simulink library "mach_lib"  (Simulink 6.3)
undefined symbols (not defined in the file): accel_cmd, aero_surf_qbar_off, aero_surf_qbar_on, altitude_stop, angular_rate_stop, att_cmd_select, att_trim_IC, att_type, att_type_numbers, bb_ellipsoid, bb_params, chi_trim_IC, command_time, compute_all_rate_cols, compute_all_vel_cols, constants, cosA, da_trim_IC, de_trim_IC, DiscIntNeverNeededParam, dr_trim_IC, dtsim, E_rwy, E_trim_IC, Ed_cmd, Ed_trim_IC, energy_stop, eow_boundary, full_surf_llim, full_surf_ulim, gain_var_struct, gam_cmd_descent, gam_cmd_preflare, gamdot_cmd_descent, gamdot_cmd_flare, gamdot_cmd_preflare, gamma_trim_IC, h_trim_IC, hd_cmd, hd_trim_IC, ideal_vel_Kb, integrate_start_time_sim, integrate_state_sim, llim, MACH, MACH_att_fb, MACH_gain_mat, MACH_mass_IC, MACH_pos_IC, MACH_pqr_Bmat_IC, MACH_pqr_IC, MACH_pqr_u_IC, MACH_quat_IC, MACH_throttle_IC, MACH_U_nom_IC, MACH_vel_Bmat_IC, MACH_vel_cvdnom_IC, MACH_vel_IC, MACH_vel_uold_IC, max_chi_cmd ... (+67)
libraries: simulink x75, mach_lib x27, utility_lib x25, model_lib x7, models x6
(part 5 of 6)

== system mach_lib/claw_main/state est/wind estimator/wind estimate ==
  note: Note: wind estimator used to assume sensed accel
      | at some (modeled) sensor location offset.
      |  Current code assumes sensed accel at CG.
  dircos : Inport
  x : Inport  Port=2
  xdot : Inport  Port=3
  model_accels_cg : Inport  Port=4
  sensed_accels_cg : Inport  Port=5
  wind_est_sw : Inport  Port=6
  Bus Creator : BusCreator  Inputs=5
  Bus Selector : BusSelector  OutputSignals=uvw
  Data Type Conversion : DataTypeConversion  OutDataTypeMode=double  SaturateOnIntegerOverflow=on  RndMeth=Zero
  Discrete-Time Integrator : DiscreteIntegrator  SampleTime=-1  ICPrevOutput=DiscIntNeverNeededParam  ICPrevScaledInput=DiscIntNeverNeededParam
  Gain : Gain  Gain=MACH.est_w_Kuvw  SaturateOnIntegerOverflow=on
  Gain1 : Gain  Orientation=left  Gain=MACH.est_w_Kaw  SaturateOnIntegerOverflow=on
  Math Function : Math  Operator=transpose  SaturateOnIntegerOverflow=on
  Product : Product  Multiplication=Matrix(*)  SaturateOnIntegerOverflow=on
  Product1 : Product  Orientation=left  Multiplication=Matrix(*)  SaturateOnIntegerOverflow=on
  Product2 : Product  SaturateOnIntegerOverflow=on
  Product3 : Product  SaturateOnIntegerOverflow=on
  Reshape : simulink/Math Operations/Reshape  OutputDimensionality=Customize  OutputDimensions=[3,3]
  Sum : Sum  Inputs=++|  SaturateOnIntegerOverflow=on  InputSameDT=on
  Sum1 : Sum  Inputs=|+-  SaturateOnIntegerOverflow=on  InputSameDT=on
  Sum2 : Sum  Inputs=-+|  SaturateOnIntegerOverflow=on
  Sum3 : Sum  Orientation=left  Inputs=-+|  SaturateOnIntegerOverflow=on
  Sum4 : Sum  Inputs=|++  SaturateOnIntegerOverflow=on  InputSameDT=on
  Unit Delay1 : UnitDelay  Orientation=left  X0=zeros(3,1)  SampleTime=-1
  rate and  position limits : Subsystem
  uvw : Selector  Elements=MACH.uvw_idx  InputPortWidth=MACH.num_x
  w_est : Outport
  w_est_debug : Outport  Port=2
  wires:
  model_accels_cg/1 -> [accels], Sum1/2
  Bus Creator/1 -> w_est_debug/1
  [accels] -> Bus Creator/5  "accels"
  [uvw_rw_est] -> Bus Creator/4  "uvw_rw_est"
  [uvw_wind] -> Bus Creator/3  "uvw_wind"
  Data Type Conversion/1 -> Product3/1, Product2/1
  Unit Delay1/1 -> Sum4/2
  Product3/1 -> Sum4/1
  Sum4/1 -> Discrete-Time Integrator/1
  wind_est_sw/1 -> Data Type Conversion/1
  Product2/1 -> Bus Creator/1, Sum3/2, w_est/1  "w_est"
  Sum3/1 -> Bus Creator/2, Product1/2  "NED_wind_ex"
  Product1/1 -> Gain1/1
  rate and  position limits/1(w_est_lim) -> Product2/2
  x/1 -> Bus Selector/1
  uvw/1 -> Sum/1
  xdot/1 -> uvw/1
  Gain1/1 -> Unit Delay1/1
  Sum2/1 -> [uvw_wind], Product/2
  Math Function/1 -> Product/1
  Product/1 -> rate and  position limits/1(w_est), Sum3/1
  Reshape/1 -> Product1/1, Math Function/1
  dircos/1 -> Reshape/1
  Bus Selector/1 -> Sum2/1  "<uvw>"
  Gain/1 -> Sum/2
  Sum/1 -> Product3/2
  Sum1/1 -> Gain/1
  sensed_accels_cg/1 -> Sum1/1
  Discrete-Time Integrator/1 -> [uvw_rw_est], Sum2/2

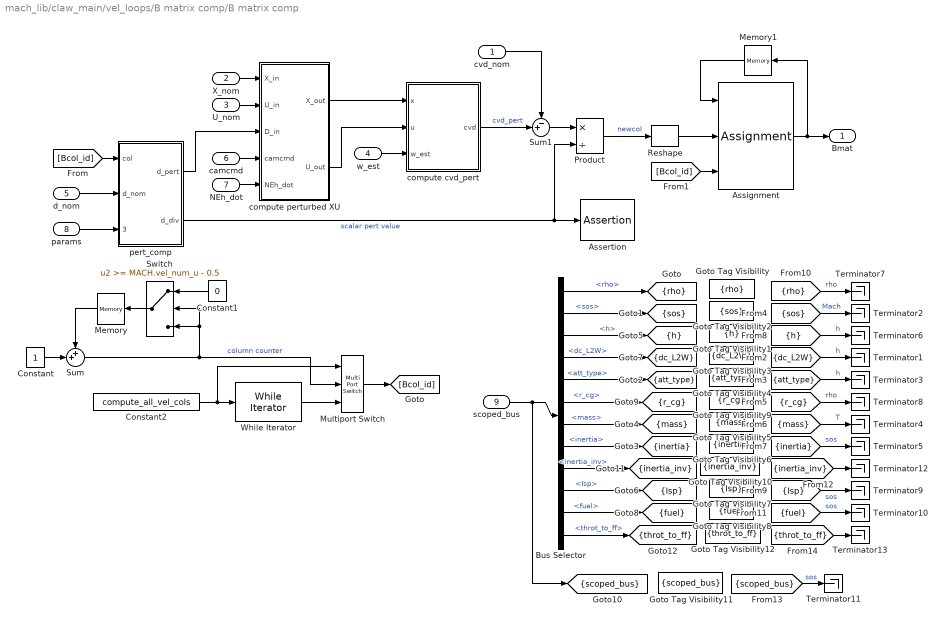
== system mach_lib/claw_main/vel_loops/B matrix comp/B matrix comp ==
  cvd_nom : Inport
  X_nom : Inport  Port=2
  U_nom : Inport  Port=3
  w_est : Inport  Port=4
  d_nom : Inport  Port=5
  camcmd : Inport  Port=6
  NEh_dot : Inport  Port=7
  params : Inport  Port=8
  scoped_bus : Inport  Port=9
  Assertion : Assertion
  Assignment : Assignment  InputType=Matrix  Rows=-1  ColumnSrc=External
  Bus Selector : BusSelector  OutputSignals=atmos_env.rho,atmos_env.sos,atmos_env.h,dc_L2W,att_type,mass_props.r_cg,mass_props.mass,mass_props.inertia,mass_props.inertia_inv,mass_props.Isp,mass_props.fuel,mass_props.throt_to_ff
  Constant : Constant
  Constant1 : Constant  Orientation=left  Value=0
  Constant2 : Constant  Value=compute_all_vel_cols
  Goto Tag Visibility : GotoTagVisibility  GotoTag=rho
  Goto Tag Visibility1 : GotoTagVisibility  GotoTag=h
  Goto Tag Visibility10 : GotoTagVisibility  GotoTag=inertia_inv
  Goto Tag Visibility11 : GotoTagVisibility  GotoTag=scoped_bus
  Goto Tag Visibility12 : GotoTagVisibility  GotoTag=throt_to_ff
  Goto Tag Visibility2 : GotoTagVisibility  GotoTag=sos
  Goto Tag Visibility3 : GotoTagVisibility  GotoTag=dc_L2W
  Goto Tag Visibility4 : GotoTagVisibility  GotoTag=att_type
  Goto Tag Visibility5 : GotoTagVisibility  GotoTag=mass
  Goto Tag Visibility6 : GotoTagVisibility  GotoTag=inertia
  Goto Tag Visibility7 : GotoTagVisibility  GotoTag=Isp
  Goto Tag Visibility8 : GotoTagVisibility  GotoTag=fuel
  Goto Tag Visibility9 : GotoTagVisibility  GotoTag=r_cg
  Memory : Memory  Orientation=left  InheritSampleTime=on
  Memory1 : Memory  Orientation=left  X0=MACH_vel_Bmat_IC  InheritSampleTime=on
  Multiport Switch : MultiPortSwitch  Inputs=2  zeroidx=on
  Product : Product  Inputs=*/  SaturateOnIntegerOverflow=on  InputSameDT=on
  Reshape : simulink/Math Operations/Reshape  OutputDimensionality=Column vector  OutputDimensions=[1,1]
  Sum : Sum  Inputs=++|  SaturateOnIntegerOverflow=on  InputSameDT=on
  Sum1 : Sum  Inputs=-+|  SaturateOnIntegerOverflow=on  InputSameDT=on
  Switch : Switch  Orientation=left  Threshold=MACH.vel_num_u - 0.5  SaturateOnIntegerOverflow=on  InputSameDT=on
  Terminator{1..13} (13 alike) : Terminator
  While Iterator : WhileIterator  MaxIters=MACH.vel_num_u  WhileBlockType=do-while  ShowIterationPort=on
  compute cvd_pert : Subsystem
  compute perturbed XU : Subsystem
  pert_comp : Subsystem
  Bmat : Outport
  tag scope: Isp=scoped, att_type=scoped, dc_L2W=scoped, fuel=scoped, h=scoped, inertia=scoped, inertia_inv=scoped, mass=scoped, r_cg=scoped, rho=scoped, scoped_bus=scoped, sos=scoped, throt_to_ff=scoped
  wires:
  [throt_to_ff] -> Terminator13/1
  Bus Selector/12 -> [throt_to_ff]  "<throt_to_ff>"
  [scoped_bus] -> Terminator11/1  "sos"
  Bus Selector/9 -> [inertia_inv]  "<inertia_inv>"
  [inertia_inv] -> Terminator12/1
  cvd_nom/1 -> Sum1/1
  compute cvd_pert/1(cvd) -> Sum1/2  "cvd_pert"
  Bus Selector/11 -> [fuel]  "<fuel>"
  [fuel] -> Terminator10/1  "sos"
  Bus Selector/10 -> [Isp]  "<Isp>"
  [Isp] -> Terminator9/1  "sos"
  Bus Selector/8 -> [inertia]  "<inertia>"
  Bus Selector/7 -> [mass]  "<mass>"
  Bus Selector/6 -> [r_cg]  "<r_cg>"
  [inertia] -> Terminator5/1  "sos"
  [mass] -> Terminator4/1  "T"
  [r_cg] -> Terminator8/1  "rho"
  Bus Selector/5 -> [att_type]  "<att_type>"
  [att_type] -> Terminator3/1  "h"
  Multiport Switch/1 -> [Bcol_id]
  Constant/1 -> Sum/2
  Memory/1 -> Sum/1
  Switch/1 -> Memory/1
  Sum/1 -> Multiport Switch/2, Switch/2, Switch/3  "column counter"
  Constant1/1 -> Switch/1
  While Iterator/1 -> Multiport Switch/3
  Constant2/1 -> While Iterator/1, Multiport Switch/1
  Bus Selector/4 -> [dc_L2W]  "<dc_L2W>"
  [dc_L2W] -> Terminator1/1  "h"
  Bus Selector/3 -> [h]  "<h>"
  Bus Selector/2 -> [sos]  "<sos>"
  Bus Selector/1 -> [rho]  "<rho>"
  [h] -> Terminator6/1  "h"
  [sos] -> Terminator2/1  "Mach"
  [rho] -> Terminator7/1  "rho"
  scoped_bus/1 -> [scoped_bus], Bus Selector/1
  Memory1/1 -> Assignment/1
  compute perturbed XU/2(U_out) -> compute cvd_pert/2(u)
  params/1 -> pert_comp/3(params)
  compute perturbed XU/1(X_out) -> compute cvd_pert/1(x)
  NEh_dot/1 -> compute perturbed XU/5(NEh_dot)
  camcmd/1 -> compute perturbed XU/4(camcmd)
  w_est/1 -> compute cvd_pert/3(w_est)
  pert_comp/1(d_pert) -> compute perturbed XU/3(D_in)
  pert_comp/2(d_div) -> Assertion/1, Product/2  "scalar pert value"
  d_nom/1 -> pert_comp/2(d_nom)
  [Bcol_id] -> pert_comp/1(col)
  Assignment/1 -> Memory1/1, Bmat/1
  Reshape/1 -> Assignment/2
  [Bcol_id] -> Assignment/3
  Sum1/1 -> Product/1
  Product/1 -> Reshape/1  "newcol"
  X_nom/1 -> compute perturbed XU/1(X_in)
  U_nom/1 -> compute perturbed XU/2(U_in)

== system mach_lib/claw_main/vel_loops/B matrix comp/compute cvd_nom ==
  note: Note: this computation of NEh accelerations
      | assumes that pqr = 0
  x : Inport
  u : Inport  Port=2
  w_est : Inport  Port=3
  Bus Selector : BusSelector  OutputSignals=dircos
  Gain : Gain  Gain=[1 1 -1]  SaturateOnIntegerOverflow=on
  Math Function : Math  Operator=transpose  SaturateOnIntegerOverflow=on
  Product : Product  Multiplication=Matrix(*)  SaturateOnIntegerOverflow=on  InputSameDT=on
  Reshape : simulink/Math Operations/Reshape  OutputDimensionality=Customize  OutputDimensions=[3,3]
  cl model : models/datcom-obac
  uvw_dot : Selector  Elements=MACH.uvw_idx  InputPortWidth=MACH.num_x
  cvd : Outport
  wires:
  cl model/2 -> Bus Selector/1
  cl model/1 -> uvw_dot/1
  w_est/1 -> cl model/3
  u/1 -> cl model/2
  Bus Selector/1 -> Reshape/1  "<dircos>"
  Gain/1 -> cvd/1
  Product/1 -> Gain/1
  Math Function/1 -> Product/1
  Reshape/1 -> Math Function/1
  x/1 -> cl model/1
  uvw_dot/1 -> Product/2

== system mach_lib/claw_main/vel_loops/B matrix comp/compute nominal XU ==
  X_in : Inport
  U_in : Inport  Port=2
  D_in : Inport  Port=3
  camcmd : Inport  Port=4
  NEh_dot : Inport  Port=5
  Assignment1 : Assignment  Elements=MACH.throttle_idx  OutputInitialize=Initialize using input (U1)
  Assignment2 : Assignment  Elements=[ MACH.quat_idx MACH.uvw_idx]  OutputInitialize=Initialize using input (U1)
  Demux1 : Demux  Outputs=[ 2 MACH.num_u_throt ]
  Gain : Gain  Gain=[1 1 -1]  SaturateOnIntegerOverflow=on
  Mux : Mux  Inputs=[ 2 1 ]
  Mux1 : Mux  Inputs=2
  Product1 : Product  Multiplication=Matrix(*)  SaturateOnIntegerOverflow=on
  Reshape1 : simulink/Math Operations/Reshape  OutputDimensionality=Customize  OutputDimensions=[3,3]
  Selector1 : Selector  Elements=MACH.quat_idx  InputPortWidth=MACH.num_x
  att2dc : utility_lib/att2dc
  dc2e_ref : utility_lib/dc2e_ref
  X_out : Outport
  U_out : Outport  Port=2
  wires:
  Mux1/1 -> Assignment2/2
  Product1/1 -> Mux1/2  "uvw"
  Selector1/1 -> dc2e_ref/2
  Gain/1 -> Product1/2  "NED_dot"
  dc2e_ref/1 -> Mux1/1  "e"
  att2dc/1 -> dc2e_ref/1, Reshape1/1
  Assignment2/1 -> X_out/1
  Reshape1/1 -> Product1/1
  NEh_dot/1 -> Gain/1
  Demux1/1 -> Mux/1
  camcmd/1 -> Mux/2
  Assignment1/1 -> U_out/1
  X_in/1 -> Selector1/1, Assignment2/1
  U_in/1 -> Assignment1/1
  D_in/1 -> Demux1/1
  Demux1/2 -> Assignment1/2  "throttle"
  Mux/1 -> att2dc/1

== system mach_lib/claw_main/vel_loops/convert accel_cmd to NED_dd_cmd/NED_dd cmd ==
  NEH_dd_cmd_in : Inport
  Action Port : ActionPort
  NEh_dd_cmd : Outport  InitialOutput=zeros(3,1)
  wires:
  NEH_dd_cmd_in/1 -> NEh_dd_cmd/1

== system mach_lib/claw_main/vel_loops/convert accel_cmd to NED_dd_cmd/vchigam_dot cmd ==
  vchigam_dot_cmd : Inport
  NEh_d : Inport  Port=2
  Action Port : ActionPort
  Math Function : Math  Operator=transpose  SaturateOnIntegerOverflow=on
  Product2 : Product  Multiplication=Matrix(*)  RndMeth=Zero
  Reshape1 : simulink/Math Operations/Reshape  OutputDimensionality=Customize  OutputDimensions=[3 3]
  convert to NED_d : Gain  Gain=[1 1 -1]
  convert to NEh_dd : Gain  Gain=[1 1 -1]
  polar to cart : Subsystem
  vec2dc : utility_lib/vec2dc
  NEh_dd_cmd : Outport  InitialOutput=zeros(3,1)
  wires:
  vec2dc/2 -> polar to cart/1(scaling_info)
  vchigam_dot_cmd/1 -> polar to cart/2(vchigam_dot_cmd)
  Math Function/1 -> Product2/1
  convert to NEh_dd/1 -> NEh_dd_cmd/1
  Product2/1 -> convert to NEh_dd/1
  NEh_d/1 -> convert to NED_d/1
  polar to cart/1(along_dd;cross_dd;vert_dd) -> Product2/2
  convert to NED_d/1 -> vec2dc/1
  Reshape1/1 -> Math Function/1
  vec2dc/1 -> Reshape1/1

== system mach_lib/claw_main/vel_loops/set di params/att limits ==
  uvw : Inport
  Bus Creator : BusCreator
  Constant : Constant  Value=MACH.vel_att_ulim  VectorParams1D=off
  Constant1 : Constant  Value=MACH.vel_att_lrlim
  Constant2 : Constant  Value=MACH.vel_att_urlim
  Constant3 : Constant  Value=MACH.az_ulim
  Constant7 : Constant  Value=MACH.vel_att_llim  VectorParams1D=off
  Constant8 : Constant  Value=MACH.az_llim
  Reshape1 : simulink/Math Operations/Reshape  OutputDimensionality=1-D array  OutputDimensions=[1,1]
  Reshape3 : simulink/Math Operations/Reshape  OutputDimensionality=1-D array  OutputDimensions=[1,1]
  Selector1 : Selector  InputType=Matrix  Elements=[1 3]  RowSrc=External  Columns=-1  InputPortWidth=3
  Selector2 : Selector  InputType=Matrix  Elements=[1 3]  RowSrc=External  Columns=-1  InputPortWidth=3
  velocity based angular rate llim : mach_lib/velocity based angular rate limit  q_idx=2
  velocity based angular rate ulim : mach_lib/velocity based angular rate limit  q_idx=2
  att_limits : Outport
  wires:
  Bus Creator/1 -> att_limits/1
  velocity based angular rate llim/1 -> Bus Creator/4  "att_lrlim"
  velocity based angular rate ulim/1 -> Bus Creator/3  "att_urlim"
  uvw/1 -> velocity based angular rate llim/3, velocity based angular rate ulim/3
  Constant3/1 -> velocity based angular rate llim/2
  Constant1/1 -> velocity based angular rate llim/1
  Constant8/1 -> velocity based angular rate ulim/2
  Constant2/1 -> velocity based angular rate ulim/1
  Reshape3/1 -> Bus Creator/2  "att_llim"
  Reshape1/1 -> Bus Creator/1  "att_ulim"
  Selector2/1 -> Reshape3/1
  Selector1/1 -> Reshape1/1
  Constant7/1 -> Selector2/1
  Constant/1 -> Selector1/1
  [att_type] -> Selector2/2, Selector1/2

== system mach_lib/claw_main/vel_loops/set di params/combine limits ==
  att_limits : Inport
  throt_limits : Inport  Port=2
  Bus Creator : BusCreator
  Bus Selector : BusSelector  OutputSignals=att_ulim,att_llim,att_urlim,att_lrlim
  Bus Selector1 : BusSelector  OutputSignals=throt_ulim,throt_llim,throt_urlim,throt_lrlim
  Mux{,1..3} (4 alike) : Mux  Inputs=2
  vel_u_limits : Outport
  wires:
  Bus Creator/1 -> vel_u_limits/1
  Mux3/1 -> Bus Creator/4  "u_lrlim"
  Mux2/1 -> Bus Creator/3  "u_urlim"
  Mux1/1 -> Bus Creator/2  "u_llim"
  Mux/1 -> Bus Creator/1  "u_ulim"
  Bus Selector1/4 -> Mux3/2  "<throt_lrlim>"
  Bus Selector1/3 -> Mux2/2  "<throt_urlim>"
  Bus Selector1/2 -> Mux1/2  "<throt_llim>"
  Bus Selector1/1 -> Mux/2  "<throt_ulim>"
  Bus Selector/4 -> Mux3/1  "<att_lrlim>"
  Bus Selector/3 -> Mux2/1  "<att_urlim>"
  Bus Selector/2 -> Mux1/1  "<att_llim>"
  Bus Selector/1 -> Mux/1  "<att_ulim>"
  throt_limits/1 -> Bus Selector1/1
  att_limits/1 -> Bus Selector/1

== system mach_lib/claw_main/vel_loops/set di params/compute dc_fltpath ==
  NEh_dot_fltpath : Inport
  Gain : Gain  Gain=repmat([1 1 -1],3,1)
  Gain1 : Gain  Gain=[1 1 -1]
  Reshape : simulink/Math Operations/Reshape  OutputDimensionality=Customize  OutputDimensions=[3 3]
  Terminator : Terminator
  vec2dc : utility_lib/vec2dc
  dc_fltpath : Outport
  wires:
  NEh_dot_fltpath/1 -> Gain1/1
  Gain/1 -> dc_fltpath/1
  vec2dc/2 -> Terminator/1
  Gain1/1 -> vec2dc/1
  Reshape/1 -> Gain/1
  vec2dc/1 -> Reshape/1

== system mach_lib/claw_main/vel_loops/set di params/throttle limits ==
  full_surf : Inport
  throt_old : Inport  Port=2
  Bus Creator : BusCreator
  Bus Selector1 : BusSelector  OutputSignals=full_surf_ulim,full_surf_llim,full_surf_urlim,full_surf_lrlim
  Selector{1..2,5..6} (4 alike) : Selector  Elements=MACH.throttle_idx  InputPortWidth=MACH.num_u
  rate limit limits : mach_lib/rate limit limits  ulim=MACH.vel_throt_ulim  llim=MACH.vel_throt_llim
  throt_limits : Outport
  wires:
  Selector2/1 -> Bus Creator/4, rate limit limits/5  "throt_lrlim"
  Selector1/1 -> Bus Creator/3, rate limit limits/4  "throt_urlim"
  Bus Selector1/4 -> Selector2/1  "<full_surf_lrlim>"
  Bus Selector1/3 -> Selector1/1  "<full_surf_urlim>"
  rate limit limits/2 -> Bus Creator/2  "throt_llim"
  rate limit limits/1 -> Bus Creator/1  "throt_ulim"
  Bus Creator/1 -> throt_limits/1
  Selector6/1 -> rate limit limits/3
  Selector5/1 -> rate limit limits/2
  throt_old/1 -> rate limit limits/1
  full_surf/1 -> Bus Selector1/1
  Bus Selector1/2 -> Selector6/1  "<full_surf_llim>"
  Bus Selector1/1 -> Selector5/1  "<full_surf_ulim>"

== system mach_lib/control input/form control input/select command/att cmd select ==
  cmd_bus : Inport
  Bus Selector1 : BusSelector  OutputSignals=att1_cmd,att2_cmd,att3_cmd,throttle_cmd  OutputAsBus=on
  Bus Selector2 : BusSelector  OutputSignals=att_cmd
  Switch : Switch  Threshold=0.5
  use_cam_rate_cmd1 : Constant  Value=att_cmd_select
  att_cmd : Outport
  wires:
  Bus Selector1/1 -> Switch/3
  Bus Selector2/1 -> Switch/1  "<att_cmd>"
  cmd_bus/1 -> Bus Selector1/1, Bus Selector2/1
  use_cam_rate_cmd1/1 -> Switch/2
  Switch/1 -> att_cmd/1

== system mach_lib/control input/form control input/select command/pos cmd select ==
  cmd_bus : Inport
  Bus Selector1 : BusSelector  OutputSignals=N_cmd,E_cmd,att3_cmd,h_cmd  OutputAsBus=on
  Bus Selector3 : BusSelector  OutputSignals=pos_cmd,accel_submode
  Bus Selector5 : BusSelector  OutputSignals=Vd_cmd,chid_cmd,att3_cmd,gammad_cmd  OutputAsBus=on
  Bus Selector6 : BusSelector  OutputSignals=Ndd_cmd,Edd_cmd,att3_cmd,hdd_cmd  OutputAsBus=on
  Constant : Constant  Value=use_NdEdh_pos
  Ground : Ground
  Multiport Switch : MultiPortSwitch  Inputs=2  zeroidx=on
  Multiport Switch1 : MultiPortSwitch  zeroidx=on
  Switch : Switch  Threshold=0.5
  convert if use_Vchigam : Subsystem
  use_cam_rate_cmd1 : Constant  Value=pos_cmd_select
  pos_cmd : Outport
  wires:
  Constant/1 -> Multiport Switch/1
  convert if use_Vchigam/1(pos_cmd) -> Multiport Switch/3
  Bus Selector1/1 -> Multiport Switch/2
  cmd_bus/1 -> Bus Selector1/1, Bus Selector6/1, Bus Selector5/1, convert if use_Vchigam/1(cmd_bus), Bus Selector3/1
  use_cam_rate_cmd1/1 -> Switch/2
  Switch/1 -> pos_cmd/1
  Bus Selector3/1 -> Switch/1  "<pos_cmd>"
  Bus Selector3/2 -> Multiport Switch1/1  "<accel_submode>"
  Multiport Switch/1 -> Multiport Switch1/2
  Ground/1 -> Multiport Switch1/5
  Bus Selector6/1 -> Multiport Switch1/3
  Bus Selector5/1 -> Multiport Switch1/4
  Multiport Switch1/1 -> Switch/3

== system mach_lib/control input/form control input/select command/rate cmd select ==
  cmd_bus : Inport
  Bus Selector1 : BusSelector  OutputSignals=p_cmd,q_cmd,r_cmd,throttle_cmd  OutputAsBus=on
  Bus Selector3 : BusSelector  OutputSignals=rate_cmd  OutputAsBus=on
  Switch : Switch  Threshold=0.5
  use_cam_rate_cmd1 : Constant  Value=rate_cmd_select
  rate_cmd : Outport
  wires:
  Switch/1 -> rate_cmd/1
  use_cam_rate_cmd1/1 -> Switch/2
  cmd_bus/1 -> Bus Selector3/1, Bus Selector1/1
  Bus Selector3/1 -> Switch/1
  Bus Selector1/1 -> Switch/3

== system mach_lib/control input/form control input/select command/vel cmd select ==
  cmd_bus : Inport
  Bus Selector1 : BusSelector  OutputSignals=Vd_cmd,chid_cmd,att3_cmd,gammad_cmd  OutputAsBus=on
  Bus Selector2 : BusSelector  OutputSignals=vel_cmd,accel_submode
  Bus Selector4 : BusSelector  OutputSignals=Ndd_cmd,Edd_cmd,att3_cmd,hdd_cmd  OutputAsBus=on
  Ground : Ground
  Multiport Switch : MultiPortSwitch  zeroidx=on
  Switch : Switch  Threshold=0.5
  convert if use_Vchigam : Subsystem
  use_cam_rate_cmd1 : Constant  Value=vel_cmd_select
  vel_cmd : Outport
  wires:
  Switch/1 -> vel_cmd/1
  use_cam_rate_cmd1/1 -> Switch/2
  cmd_bus/1 -> Bus Selector2/1, Bus Selector4/1, Bus Selector1/1, convert if use_Vchigam/1(cmd_bus)
  Bus Selector2/1 -> Switch/1  "<vel_cmd>"
  Bus Selector2/2 -> Multiport Switch/1  "<accel_submode>"
  Bus Selector4/1 -> Multiport Switch/3
  Ground/1 -> Multiport Switch/5
  Bus Selector1/1 -> Multiport Switch/4
  Multiport Switch/1 -> Switch/3
  convert if use_Vchigam/1(vel_cmd) -> Multiport Switch/2

== system mach_lib/control input/generate commands/pos cmd generator/circle pos cmd ==
  cmd_bus : Inport
  Bus Selector1 : BusSelector  OutputSignals=att3_cmd,h_cmd  OutputAsBus=on
  Constant : Constant
  Gain : Gain  Gain=50
  Gain1 : Gain  Gain=50
  Gain2 : Gain  Gain=0.1
  Gain3 : Gain
  Mux1 : Mux  Inputs=3
  Ramp : Subsystem  mask{slope=1, start_time=command_time, initial_output=0, sample_time=MACH.dt}
      mask prompts: start_time "Start time:"; initial_output "Initial output:"; sample_time "Sample time (-1 for inherited):"
  Saturation1 : Saturate  UpperLimit=10  LowerLimit=0
  Sum : Sum  Inputs=|-+
  Sum1 : Sum  Inputs=++|
  Sum2 : Sum  Inputs=-+|
  Trigonometric Function : Trigonometry
  Trigonometric Function1 : Trigonometry  Operator=cos
  pos_cmd : Outport
  wires:
  Sum/1 -> Gain1/1
  Trigonometric Function/1 -> Gain/1
  Sum2/1 -> Gain2/1
  Trigonometric Function1/1 -> Sum/1
  Constant/1 -> Sum/2
  Gain1/1 -> Mux1/2
  Sum1/1 -> Mux1/1
  Gain/1 -> Sum1/2
  Ramp/1(ramp) -> Saturation1/1, Sum2/2
  Saturation1/1 -> Sum2/1, Gain3/1
  Gain2/1 -> Trigonometric Function/1, Trigonometric Function1/1
  Gain3/1 -> Sum1/1
  cmd_bus/1 -> Bus Selector1/1
  Bus Selector1/1 -> Mux1/3
  Mux1/1 -> pos_cmd/1

== system mach_lib/control input/generate commands/pos cmd generator/ramp pos cmd ==
  cmd_bus : Inport
  Bus Selector1 : BusSelector  OutputSignals=E_cmd,att3_cmd,h_cmd  OutputAsBus=on
  Discrete-Time Integrator1 : DiscreteIntegrator  SampleTime=-1  ICPrevOutput=DiscIntNeverNeededParam  ICPrevScaledInput=DiscIntNeverNeededParam
  Discrete-Time Integrator3 : DiscreteIntegrator  SampleTime=-1  ICPrevOutput=DiscIntNeverNeededParam  ICPrevScaledInput=DiscIntNeverNeededParam
  Gain : Gain  Gain=ideal_vel_Kb
  Mux : Mux  Inputs=2
  Sum6 : Sum  Inputs=|+-  SaturateOnIntegerOverflow=on
  limit acceleration to g/3 : Saturate  UpperLimit=constants.g/3  LowerLimit=-constants.g/3
  velocity command : Step  Time=command_time  After=1.69*15  SampleTime=MACH.dt
  pos_cmd : Outport
  wires:
  limit acceleration to g/3/1 -> Discrete-Time Integrator3/1
  Gain/1 -> limit acceleration to g/3/1
  Sum6/1 -> Gain/1
  velocity command/1 -> Sum6/1
  Discrete-Time Integrator3/1 -> Discrete-Time Integrator1/1, Sum6/2
  Discrete-Time Integrator1/1 -> Mux/1
  Mux/1 -> pos_cmd/1
  cmd_bus/1 -> Bus Selector1/1
  Bus Selector1/1 -> Mux/2

== system mach_lib/control input/generate commands/vel cmd generator/Ramp ==
  From Workspace1 : FromWorkspace  VariableName=[ 0 initial_output ; start_time initial_output ; start_time+1 initial_output+slope ]  SampleTime=MACH.dt
  ramp : Outport
  wires:
  From Workspace1/1 -> ramp/1

== system mach_lib/control input/generate commands/vel cmd generator/descent ==
  From Workspace1 : FromWorkspace  VariableName=[ 0 initial_output ; start_time initial_output ; start_time+1 initial_output+slope ]  SampleTime=MACH.dt
  ramp : Outport
  wires:
  From Workspace1/1 -> ramp/1

== system mach_lib/control input/generate commands/vel cmd generator/flare ==
  From Workspace1 : FromWorkspace  VariableName=[ 0 initial_output ; start_time initial_output ; start_time+1 initial_output+slope ]  SampleTime=MACH.dt
  ramp : Outport
  wires:
  From Workspace1/1 -> ramp/1

== system mach_lib/control input/generate commands/vel cmd generator/pre-flare ==
  From Workspace1 : FromWorkspace  VariableName=[ 0 initial_output ; start_time initial_output ; start_time+1 initial_output+slope ]  SampleTime=MACH.dt
  ramp : Outport
  wires:
  From Workspace1/1 -> ramp/1

== system mach_lib/control input/generate commands/vel cmd generator/turn rate ==
  From Workspace1 : FromWorkspace  VariableName=[ 0 initial_output ; start_time initial_output ; start_time+1 initial_output+slope ]  SampleTime=MACH.dt
  ramp : Outport
  wires:
  From Workspace1/1 -> ramp/1

== system mach_lib/claw_main/input processing/mode dependent stick processing/att rate cmd/also reset att on att_type change ==
  reset_in : Inport
  Detect Change : simulink/Logic and Bit Operations/Detect Change  vinit=0
  Detect Increase : simulink/Logic and Bit Operations/Detect Increase  vinit=0.0
  Logical Operator2 : Logic  Operator=OR  AllPortsSameDT=off
  Logical Operator3 : Logic  Operator=XOR  AllPortsSameDT=off
  Unit Delay : UnitDelay  Orientation=left  SampleTime=MACH.dt
  reset_out : Outport
  wires:
  reset_in/1 -> Detect Increase/1
  Unit Delay/1 -> Logical Operator3/2
  Logical Operator3/1 -> reset_out/1, Unit Delay/1
  Logical Operator2/1 -> Logical Operator3/1
  Detect Increase/1 -> Logical Operator2/1
  Detect Change/1 -> Logical Operator2/2
  [att_type] -> Detect Change/1

== system mach_lib/claw_main/input processing/mode dependent stick processing/feed forward/get att_ff ==
  signal_bus : Inport
  Bus Selector : BusSelector  OutputSignals=x_est.uvw,y_meas.accels_cg,y_meas.dircos,x_est.e
  Dot Product : simulink/Math Operations/Dot Product  InputSameDT=on  OutDataType=sfix(16)  OutScaling=2^-10  DoSatur=off
  Gain : Gain  Gain=constants.g
  MinMax1 : MinMax  Function=max  Inputs=2
  Product1 : Product  Inputs=/*  RndMeth=Zero
  Sum2 : Sum  Inputs=|++
  V x a : utility_lib/cross product
  down vector : Selector  Elements=7:9  InputPortWidth=9
  geted : utility_lib/geted
  protect for   divide by zero : Constant  Value=0.001^2
  att_ff : Outport
  wires:
  Dot Product/1 -> MinMax1/1
  Bus Selector/2 -> Sum2/1  "<accels_cg>"
  Gain/1 -> Sum2/2
  down vector/1 -> Gain/1
  Bus Selector/3 -> down vector/1  "<dircos>"
  geted/1 -> att_ff/1
  Sum2/1 -> V x a/2
  MinMax1/1 -> Product1/1
  protect for   divide by zero/1 -> MinMax1/2
  Bus Selector/4 -> geted/2  "<e>"
  Bus Selector/1 -> Dot Product/2, Dot Product/1, V x a/1  "<uvw>"
  signal_bus/1 -> Bus Selector/1
  V x a/1 -> Product1/2
  Product1/1 -> geted/1

== system mach_lib/claw_main/input processing/mode dependent stick processing/feed forward/lookup using  energy over weight ==
  eow_idx : Inport
  Constant1 : Constant  Value=int32(0:2)
  Constant2 : Constant  Value=int32(0:2)
  Interpolation (n-D) using PreLookup for acc : simulink/Lookup Tables/Interpolation (n-D) using PreLookup  numDimsPopupSelect=2  explicitNumDims=2  table=tbl_acc_eow  interpMethod=Linear  extrapMethod=Linear  rangeErrorMode=None  NumSelectionDims=1
  Interpolation (n-D) using PreLookup for vel : simulink/Lookup Tables/Interpolation (n-D) using PreLookup  numDimsPopupSelect=2  explicitNumDims=2  table=tbl_vel_eow  interpMethod=Linear  extrapMethod=Linear  rangeErrorMode=None  NumSelectionDims=1
  pos_ff : Outport
  vel_ff : Outport  Port=2
  wires:
  Constant2/1 -> Interpolation (n-D) using PreLookup for acc/2
  Constant1/1 -> Interpolation (n-D) using PreLookup for vel/2
  eow_idx/1 -> Interpolation (n-D) using PreLookup for acc/1, Interpolation (n-D) using PreLookup for vel/1
  Interpolation (n-D) using PreLookup for acc/1 -> vel_ff/1
  Interpolation (n-D) using PreLookup for vel/1 -> pos_ff/1

== system mach_lib/claw_main/input processing/mode dependent stick processing/feed forward/lookup using X   ==
  X_idx : Inport
  Constant1 : Constant  Value=int32(0:2)
  Constant2 : Constant  Value=int32(0:2)
  Interpolation (n-D) using PreLookup for acc : simulink/Lookup Tables/Interpolation (n-D) using PreLookup  numDimsPopupSelect=2  explicitNumDims=2  table=tbl_acc_X  interpMethod=Linear  extrapMethod=Linear  rangeErrorMode=None  NumSelectionDims=1
  Interpolation (n-D) using PreLookup for vel : simulink/Lookup Tables/Interpolation (n-D) using PreLookup  numDimsPopupSelect=2  explicitNumDims=2  table=tbl_vel_X  interpMethod=Linear  extrapMethod=Linear  rangeErrorMode=None  NumSelectionDims=1
  pos_ff : Outport
  vel_ff : Outport  Port=2
  wires:
  Constant2/1 -> Interpolation (n-D) using PreLookup for acc/2
  Constant1/1 -> Interpolation (n-D) using PreLookup for vel/2
  Interpolation (n-D) using PreLookup for acc/1 -> vel_ff/1
  Interpolation (n-D) using PreLookup for vel/1 -> pos_ff/1
  X_idx/1 -> Interpolation (n-D) using PreLookup for acc/1, Interpolation (n-D) using PreLookup for vel/1

== system mach_lib/claw_main/input processing/mode dependent stick processing/set command selection switches/modify for accel cmd submode ==
  select_cmd_in : Inport
  accel_cmd_sw : Inport  Port=2
  Assignment : Assignment  Elements=[1 2 4]  OutputInitialize=Initialize using input (U1)
  Assignment1 : Assignment  Elements=[1 2 4]  OutputInitialize=Initialize using input (U1)
  Bus Assignment : BusAssignment  AssignedSignals=vel,pos
  Bus Selector : BusSelector  OutputSignals=vel
  Bus Selector1 : BusSelector  OutputSignals=pos
  Selector1 : Selector  Elements=[1 2 4]  InputPortWidth=4
  Selector2 : Selector  Elements=[1 2 4]  InputPortWidth=4
  Switch : Switch  Threshold=0.5
  Switch1 : Switch  Threshold=0.5
  command current pos : Constant  Value=0
  command current vel : Constant  Value=0
  select_cmd : Outport
  wires:
  Assignment1/1 -> Bus Assignment/3
  Switch1/1 -> Assignment1/2
  Selector2/1 -> Switch1/3
  command current pos/1 -> Switch1/1
  Bus Selector1/1 -> Assignment1/1, Selector2/1  "<pos>"
  Bus Assignment/1 -> select_cmd/1
  Assignment/1 -> Bus Assignment/2
  Switch/1 -> Assignment/2
  Selector1/1 -> Switch/3
  command current vel/1 -> Switch/1
  Bus Selector/1 -> Assignment/1, Selector1/1  "<vel>"
  accel_cmd_sw/1 -> Switch1/2, Switch/2
  select_cmd_in/1 -> Bus Selector1/1, Bus Selector/1, Bus Assignment/1

== system mach_lib/claw_main/input processing/mode dependent stick processing/use table lookup pos cmds/use E/W to get pos cmds ==
  eow_idx : Inport
  Constant1 : Constant  Value=int32(0:2)
  Interpolation (n-D) using PreLookup : simulink/Lookup Tables/Interpolation (n-D) using PreLookup  numDimsPopupSelect=2  explicitNumDims=2  table=tbl_pos_eow  interpMethod=Linear  extrapMethod=Linear  rangeErrorMode=None  NumSelectionDims=1
  pos_cmd_eow : Outport
  wires:
  Constant1/1 -> Interpolation (n-D) using PreLookup/2
  eow_idx/1 -> Interpolation (n-D) using PreLookup/1
  Interpolation (n-D) using PreLookup/1 -> pos_cmd_eow/1

== system mach_lib/claw_main/input processing/mode dependent stick processing/use table lookup pos cmds/use X to get pos cmds ==
  note: Note: When X is used as the independent variable
      | the trajectory is in a vertical plane and Y=0
  X_idx : Inport
  X : Inport  Port=2
  Constant1 : Constant  Value=E_rwy
  Constant3 : Constant  Value=N_rwy
  Constant4 : Constant  Value=cosA
  Constant5 : Constant  Value=sinA
  Interpolation (n-D) using PreLookup for h : simulink/Lookup Tables/Interpolation (n-D) using PreLookup  numDimsPopupSelect=1  explicitNumDims=2  table=tbl_hofX  interpMethod=Linear  extrapMethod=Linear  rangeErrorMode=None  NumSelectionDims=0
  Mux : Mux  Inputs=3
  Product3 : Product  RndMeth=Zero
  Product4 : Product  RndMeth=Zero
  Sum4 : Sum  Inputs=++|
  Sum5 : Sum  Inputs=|++
  pos_cmd_X : Outport
  wires:
  X/1 -> Product3/2, Product4/2
  Constant1/1 -> Sum5/2
  Product3/1 -> Sum5/1
  Sum5/1 -> Mux/2
  Constant3/1 -> Sum4/1
  Product4/1 -> Sum4/2
  Sum4/1 -> Mux/1
  Constant5/1 -> Product3/1
  Constant4/1 -> Product4/1
  Mux/1 -> pos_cmd_X/1
  Interpolation (n-D) using PreLookup for h/1 -> Mux/3
  X_idx/1 -> Interpolation (n-D) using PreLookup for h/1

== system mach_lib/claw_main/input processing/set control parameters/accel submode setup/NED_dd/vchigam_dot ==
  case : Inport
  signal_bus : Inport  Port=2
  Action Port : ActionPort
  Bus Selector3 : BusSelector  OutputSignals=cmd_bus.autopilot_cmd
  Gain : Gain  Gain=[1 1 1]
  Selector : Selector  Elements=[1 2 4]  InputPortWidth=4
  Signal Conversion : SignalConversion  ConversionOutput=Contiguous copy
  accel_cmd_sw : Outport  InitialOutput=zeros(3,1)
  accel_cmd : Outport  Port=2  InitialOutput=zeros(3,1)
  wires:
  Signal Conversion/1 -> accel_cmd/1
  Gain/1 -> accel_cmd_sw/1
  case/1 -> Gain/1
  Selector/1 -> Signal Conversion/1
  Bus Selector3/1 -> Selector/1  "<autopilot_cmd>"
  signal_bus/1 -> Bus Selector3/1

== system mach_lib/claw_main/input processing/set control parameters/accel submode setup/homing ==
  signal_bus : Inport
  Action Port : ActionPort
  Bus Selector3 : BusSelector  OutputSignals=y_meas.seeker.aux_info.Rslant,y_meas.seeker.LOS_rate
  Compare To Constant : simulink/Logic and Bit Operations/Compare To Constant  relop=<=  const=target_range_homing  LogicOutDataTypeMode=boolean  ZeroCross=off
  Compare To Constant1 : simulink/Logic and Bit Operations/Compare To Constant  relop=<=  const=target_range_detect  LogicOutDataTypeMode=boolean  ZeroCross=off
  Compare To Constant2 : simulink/Logic and Bit Operations/Compare To Constant  relop=>=  const=target_range_blind  LogicOutDataTypeMode=boolean  ZeroCross=off
  Constant2 : Constant  Value=0
  Data Type Conversion : DataTypeConversion  OutDataTypeMode=double
  Gain : Gain  Gain=2
  Logical Operator2 : Logic  AllPortsSameDT=off
  Mux : Mux  Inputs=2
  Mux1 : Mux  Inputs=2
  Product3 : Product  RndMeth=Zero
  Selector3 : Selector  Elements=[1 1 2]  InputPortWidth=2
  azimuth_d/elevation_d gain : Gain  Gain=MACH.K_pn
  accel_cmd_sw : Outport  InitialOutput=zeros(3,1)
  accel_cmd : Outport  Port=2  InitialOutput=zeros(3,1)
  wires:
  Data Type Conversion/1 -> Gain/1
  Mux1/1 -> accel_cmd/1
  Gain/1 -> accel_cmd_sw/1
  azimuth_d/elevation_d gain/1 -> Mux1/2
  Constant2/1 -> Mux1/1
  Logical Operator2/1 -> Product3/1  "PN_active"
  Product3/1 -> azimuth_d/elevation_d gain/1
  Bus Selector3/2 -> Product3/2  "<LOS_rate>"
  signal_bus/1 -> Bus Selector3/1
  Selector3/1 -> Data Type Conversion/1
  Compare To Constant2/1 -> Logical Operator2/2
  Mux/1 -> Selector3/1, Logical Operator2/1
  Compare To Constant/1 -> Mux/2
  Compare To Constant1/1 -> Mux/1
  Bus Selector3/1 -> Compare To Constant2/1, Compare To Constant1/1, Compare To Constant/1  "<Rslant>"

== system mach_lib/claw_main/input processing/set control parameters/accel submode setup/normal vel desdyn ==
  Action Port : ActionPort
  Constant1 : Constant  Value=zeros(3,1)
  Constant2 : Constant  Value=zeros(3,1)
  accel_cmd_sw : Outport  InitialOutput=zeros(3,1)
  accel_cmd : Outport  Port=2  InitialOutput=zeros(3,1)
  wires:
  Constant2/1 -> accel_cmd_sw/1
  Constant1/1 -> accel_cmd/1

== system mach_lib/claw_main/input processing/set control parameters/select gains/mux to bus ==
  mux_in : Inport
  Bus Creator : BusCreator  Inputs=16
  Demux : Demux  Outputs=[4;4;4;4;3;3;3;3;3;3;3;3;3;3;3;3]
  bus_out : Outport
  wires:
  Demux/16 -> Bus Creator/16  "MACH_vel_Ki"
  Demux/15 -> Bus Creator/15  "MACH_vel_Kf"
  Demux/14 -> Bus Creator/14  "MACH_vel_Kb"
  Demux/13 -> Bus Creator/13  "MACH_vel_Kaw"
  Demux/12 -> Bus Creator/12  "MACH_pqr_Ki"
  Demux/11 -> Bus Creator/11  "MACH_pqr_Kf"
  Demux/10 -> Bus Creator/10  "MACH_pqr_Kb"
  Demux/9 -> Bus Creator/9  "MACH_pqr_Kaw"
  Demux/8 -> Bus Creator/8  "MACH_pos_Ki"
  Demux/7 -> Bus Creator/7  "MACH_pos_Kf"
  Demux/6 -> Bus Creator/6  "MACH_pos_Kb"
  Demux/5 -> Bus Creator/5  "MACH_pos_Kaw"
  Demux/4 -> Bus Creator/4  "MACH_att_Ki"
  Demux/3 -> Bus Creator/3  "MACH_att_Kf"
  Demux/2 -> Bus Creator/2  "MACH_att_Kb"
  Demux/1 -> Bus Creator/1  "MACH_att_Kaw"
  Bus Creator/1 -> bus_out/1
  mux_in/1 -> Demux/1

== system mach_lib/claw_main/input processing/set control parameters/set rate di params/fix aero surfs when low qbar ==
  pqr_u_ulim_in : Inport
  pqr_u_llim_in : Inport  Port=2
  low_qbar : Inport  Port=3
  pqr_u_pref : Inport  Port=4
  Assignment : Assignment  Elements=MACH.vane_idx  OutputInitialize=Initialize using input (U1)
  Assignment1 : Assignment  Elements=MACH.vane_idx  OutputInitialize=Initialize using input (U1)
  MinMax : MinMax  Inputs=2
  MinMax1 : MinMax  Function=max  Inputs=2
  Multiport Switch1 : MultiPortSwitch  Inputs=2  zeroidx=on  SaturateOnIntegerOverflow=on
  Multiport Switch2 : MultiPortSwitch  Inputs=2  zeroidx=on  SaturateOnIntegerOverflow=on
  Selector1 : Selector  Elements=MACH.vane_idx  InputPortWidth=MACH.pqr_num_u
  Selector2 : Selector  Elements=MACH.vane_idx  InputPortWidth=MACH.pqr_num_u
  Selector6 : Selector  Elements=MACH.vane_idx  InputPortWidth=MACH.pqr_num_u
  pqr_u_ulim : Outport
  pqr_u_llim : Outport  Port=2
  wires:
  MinMax1/1 -> Assignment1/2, Assignment/2
  Selector2/1 -> MinMax1/2
  MinMax/1 -> MinMax1/1
  Selector6/1 -> MinMax/2
  Selector1/1 -> MinMax/1
  Assignment1/1 -> Multiport Switch2/3
  Multiport Switch2/1 -> pqr_u_llim/1
  Assignment/1 -> Multiport Switch1/3
  Multiport Switch1/1 -> pqr_u_ulim/1
  pqr_u_llim_in/1 -> Selector2/1, Multiport Switch2/2, Assignment1/1
  pqr_u_ulim_in/1 -> Selector1/1, Multiport Switch1/2, Assignment/1
  pqr_u_pref/1 -> Selector6/1
  low_qbar/1 -> Multiport Switch2/1, Multiport Switch1/1

== system mach_lib/claw_main/input processing/set control parameters/set rate di params/select u_pref ==
  note: Use schedule if configured and qbar is low
  note: "test" not yet implemented
  note: "from outer" not yet implemented
  low_qbar : Inport
  aero_env_est : Inport  Port=2
  full_surf : Inport  Port=3
  Bus Selector4 : BusSelector  OutputSignals=full_surf_pref_select,full_surf_pref,full_surf_pref_wght,full_surf_cmd
  Constant2 : Constant  Value=MACH.pqr_wght_u_pref_high
  Demux : Demux  Outputs=2
  From Workspace : FromWorkspace  VariableName=use_preference_schedule_fw  SampleTime=MACH.dt  Interpolate=off  OutputAfterFinalValue=Holding final value
  Logical Operator : Logic  AllPortsSameDT=off
  Logical Operator1 : Logic  Operator=NOT  AllPortsSameDT=off
  MinMax : MinMax  Function=max  Inputs=2
  Multiport Switch : MultiPortSwitch  Inputs=5  zeroidx=on
  Mux{,1..3} (4 alike) : Mux  Inputs=2
  Selector{1..3,5} (4 alike) : Selector  Elements=MACH.pqr_u_idx  InputPortWidth=MACH.num_u
  preference schedule : models/BF preference schedule
  u_pref : Outport
  wght_u_pref : Outport  Port=2
  wires:
  Logical Operator/1 -> MinMax/1
  From Workspace/1 -> Logical Operator/1
  Logical Operator1/1 -> Logical Operator/2
  MinMax/1 -> Mux3/2, Mux3/1
  Mux3/1 -> Multiport Switch/1
  Selector3/1 -> MinMax/2
  Bus Selector4/4 -> Selector5/1  "<full_surf_cmd>"
  Bus Selector4/3 -> Selector2/1  "<full_surf_pref_wght>"
  Bus Selector4/2 -> Selector1/1  "<full_surf_pref>"
  Bus Selector4/1 -> Selector3/1  "<full_surf_pref_select>"
  Selector5/1 -> Mux2/1
  Constant2/1 -> Mux2/2
  Mux2/1 -> Multiport Switch/4
  full_surf/1 -> Bus Selector4/1
  low_qbar/1 -> Logical Operator1/1
  Mux1/1 -> Multiport Switch/3
  preference schedule/2 -> Mux1/2
  preference schedule/1 -> Mux1/1
  aero_env_est/1 -> preference schedule/3
  Demux/2 -> wght_u_pref/1
  Demux/1 -> u_pref/1
  Multiport Switch/1 -> Demux/1
  Mux/1 -> Multiport Switch/6, Multiport Switch/5, Multiport Switch/2
  Selector2/1 -> Mux/2, preference schedule/2
  Selector1/1 -> Mux/1, preference schedule/1

== system mach_lib/claw_main/state est/wind estimator/wind estimate/rate and  position limits ==
  w_est : Inport
  Constant : Constant  Value=MACH.est_w_ulim
  Constant1 : Constant  Value=MACH.est_w_llim
  Constant2 : Constant  Value=MACH.est_w_urlim
  Constant3 : Constant  Value=MACH.est_w_lrlim
  MinMax : MinMax  Function=max  Inputs=2  SaturateOnIntegerOverflow=on  InputSameDT=on
  MinMax1 : MinMax  Inputs=2  SaturateOnIntegerOverflow=on  InputSameDT=on
  Unit Delay : UnitDelay  SampleTime=-1
  limit computation : mach_lib/limit computation
  w_est_lim : Outport
  wires:
  Constant3/1 -> limit computation/5
  limit computation/2 -> MinMax/2
  MinMax/1 -> Unit Delay/1, w_est_lim/1
  Constant2/1 -> limit computation/4
  Constant1/1 -> limit computation/2
  Constant/1 -> limit computation/3
  limit computation/1 -> MinMax1/2
  MinMax1/1 -> MinMax/1
  Unit Delay/1 -> limit computation/1
  w_est/1 -> MinMax1/1

== system mach_lib/claw_main/vel_loops/B matrix comp/B matrix comp/compute cvd_pert ==
  note: Note: this computation of NEh accelerations
      | assumes that pqr = 0
  x : Inport
  u : Inport  Port=2
  w_est : Inport  Port=3
  Bus Selector : BusSelector  OutputSignals=dircos
  Gain : Gain  Gain=[1 1 -1]  SaturateOnIntegerOverflow=on
  Math Function : Math  Operator=transpose  SaturateOnIntegerOverflow=on
  Product : Product  Multiplication=Matrix(*)  SaturateOnIntegerOverflow=on  InputSameDT=on
  Reshape : simulink/Math Operations/Reshape  OutputDimensionality=Customize  OutputDimensions=[3,3]
  cl model : models/datcom-obac
  uvw_dot : Selector  Elements=MACH.uvw_idx  InputPortWidth=MACH.num_x
  cvd : Outport
  wires:
  cl model/2 -> Bus Selector/1
  cl model/1 -> uvw_dot/1
  w_est/1 -> cl model/3
  u/1 -> cl model/2
  Bus Selector/1 -> Reshape/1  "<dircos>"
  Gain/1 -> cvd/1
  Product/1 -> Gain/1
  Math Function/1 -> Product/1
  Reshape/1 -> Math Function/1
  x/1 -> cl model/1
  uvw_dot/1 -> Product/2

== system mach_lib/claw_main/vel_loops/B matrix comp/B matrix comp/compute perturbed XU ==
  X_in : Inport
  U_in : Inport  Port=2
  D_in : Inport  Port=3
  camcmd : Inport  Port=4
  NEh_dot : Inport  Port=5
  Assignment1 : Assignment  Elements=MACH.throttle_idx  OutputInitialize=Initialize using input (U1)
  Assignment2 : Assignment  Elements=[ MACH.quat_idx MACH.uvw_idx]  OutputInitialize=Initialize using input (U1)
  Demux1 : Demux  Outputs=[ 2 MACH.num_u_throt ]
  Gain : Gain  Gain=[1 1 -1]  SaturateOnIntegerOverflow=on
  Mux : Mux  Inputs=[ 2 1 ]
  Mux1 : Mux  Inputs=2
  Product1 : Product  Multiplication=Matrix(*)  SaturateOnIntegerOverflow=on
  Reshape1 : simulink/Math Operations/Reshape  OutputDimensionality=Customize  OutputDimensions=[3,3]
  Selector1 : Selector  Elements=MACH.quat_idx  InputPortWidth=MACH.num_x
  att2dc : utility_lib/att2dc
  dc2e_ref : utility_lib/dc2e_ref
  X_out : Outport
  U_out : Outport  Port=2
  wires:
  Mux1/1 -> Assignment2/2
  Product1/1 -> Mux1/2  "uvw"
  Selector1/1 -> dc2e_ref/2
  Gain/1 -> Product1/2  "NED_dot"
  dc2e_ref/1 -> Mux1/1  "e"
  att2dc/1 -> dc2e_ref/1, Reshape1/1
  Assignment2/1 -> X_out/1
  Reshape1/1 -> Product1/1
  NEh_dot/1 -> Gain/1
  Demux1/1 -> Mux/1
  camcmd/1 -> Mux/2
  Assignment1/1 -> U_out/1
  X_in/1 -> Selector1/1, Assignment2/1
  U_in/1 -> Assignment1/1
  D_in/1 -> Demux1/1
  Demux1/2 -> Assignment1/2  "throttle"
  Mux/1 -> att2dc/1

== system mach_lib/claw_main/vel_loops/B matrix comp/B matrix comp/pert_comp ==
  col : Inport
  d_nom : Inport  Port=2
  params : Inport  Port=3
  Bus Selector : BusSelector  OutputSignals=u_ulim,u_llim
  Constant2 : Constant  Value=diag(MACH.vel_u_pert)
  pick +/- pert : mach_lib/pick +//- pert  num_u=MACH.vel_num_u
  d_pert : Outport
  d_div : Outport  Port=2
  wires:
  Bus Selector/2 -> pick +/- pert/4  "<u_llim>"
  Bus Selector/1 -> pick +/- pert/3  "<u_ulim>"
  params/1 -> Bus Selector/1
  Constant2/1 -> pick +/- pert/5
  col/1 -> pick +/- pert/1
  pick +/- pert/1 -> d_pert/1
  d_nom/1 -> pick +/- pert/2
  pick +/- pert/2 -> d_div/1  "scalar pert value"

== system mach_lib/claw_main/vel_loops/convert accel_cmd to NED_dd_cmd/vchigam_dot cmd/polar to cart ==
  note: Note: these are actually Vground and Vslant
  scaling_info : Inport
  vchigam_dot_cmd : Inport  Port=2
  Bus Selector : BusSelector  OutputSignals=Rground,Rslant
  Demux : Demux  Outputs=[1 2]
  Gain1 : Gain  Gain=[1 -1]
  Mux : Mux  Inputs=2
  Mux1 : Mux  Inputs=2
  Product3 : Product  RndMeth=Zero
  along_dd;cross_dd;vert_dd : Outport
  wires:
  Mux1/1 -> along_dd;cross_dd;vert_dd/1
  Product3/1 -> Mux1/2
  Demux/1 -> Mux1/1
  Demux/2 -> Product3/1
  Gain1/1 -> Product3/2
  Bus Selector/2 -> Mux/2  "<Rslant>"
  Bus Selector/1 -> Mux/1  "<Rground>"
  vchigam_dot_cmd/1 -> Demux/1
  Mux/1 -> Gain1/1
  scaling_info/1 -> Bus Selector/1

== system mach_lib/control input/form control input/select command/pos cmd select/convert if use_Vchigam ==
  cmd_bus : Inport
  Bus Assignment : BusAssignment  AssignedSignals=Nd_cmd,Ed_cmd
  Bus Selector3 : BusSelector  OutputSignals=Nd_cmd,Ed_cmd,att3_cmd,h_cmd  OutputAsBus=on
  Bus Selector5 : BusSelector  OutputSignals=V_cmd,chi_cmd,use_Vchigam
  Constant : Constant  Value=0
  Switch : Switch  Threshold=0.5
  Terminator : Terminator
  vchigam2NdEdhd : utility_lib/vchigam2NdEdhd
  pos_cmd : Outport
  wires:
  cmd_bus/1 -> Bus Selector5/1, Bus Selector3/1
  vchigam2NdEdhd/1 -> Bus Assignment/2
  vchigam2NdEdhd/2 -> Bus Assignment/3
  vchigam2NdEdhd/3 -> Terminator/1
  Bus Selector5/1 -> vchigam2NdEdhd/1  "<V_cmd>"
  Bus Selector3/1 -> Bus Assignment/1, Switch/3
  Bus Selector5/3 -> Switch/2  "<use_Vchigam>"
  Bus Assignment/1 -> Switch/1
  Switch/1 -> pos_cmd/1
  Bus Selector5/2 -> vchigam2NdEdhd/2  "<chi_cmd>"
  Constant/1 -> vchigam2NdEdhd/3

== system mach_lib/control input/form control input/select command/vel cmd select/convert if use_Vchigam ==
  cmd_bus : Inport
  Bus Assignment : BusAssignment  AssignedSignals=Nd_cmd,Ed_cmd,hd_cmd
  Bus Selector3 : BusSelector  OutputSignals=Nd_cmd,Ed_cmd,att3_cmd,hd_cmd  OutputAsBus=on
  Bus Selector5 : BusSelector  OutputSignals=V_cmd,chi_cmd,gamma_cmd,use_Vchigam
  Switch : Switch  Threshold=0.5
  vchigam2NdEdhd : utility_lib/vchigam2NdEdhd
  vel_cmd : Outport
  wires:
  cmd_bus/1 -> Bus Selector5/1, Bus Selector3/1
  vchigam2NdEdhd/1 -> Bus Assignment/2
  vchigam2NdEdhd/2 -> Bus Assignment/3
  vchigam2NdEdhd/3 -> Bus Assignment/4
  Bus Selector5/1 -> vchigam2NdEdhd/1  "<V_cmd>"
  Bus Selector5/2 -> vchigam2NdEdhd/2  "<chi_cmd>"
  Bus Selector5/3 -> vchigam2NdEdhd/3  "<gamma_cmd>"
  Bus Selector3/1 -> Bus Assignment/1, Switch/3
  Bus Selector5/4 -> Switch/2  "<use_Vchigam>"
  Bus Assignment/1 -> Switch/1
  Switch/1 -> vel_cmd/1

== system mach_lib/control input/generate commands/pos cmd generator/circle pos cmd/Ramp ==
  From Workspace1 : FromWorkspace  VariableName=[ 0 initial_output ; start_time initial_output ; start_time+1 initial_output+slope ]  SampleTime=MACH.dt
  ramp : Outport
  wires:
  From Workspace1/1 -> ramp/1

== matlab function claw_main/rate_loops/allocation/RCS allocation/Embedded MATLAB Function ==
  data: Bmat input inherited; wght_cv input inherited; ulim input inherited; llim input inherited; cvd_des input inherited; rcs_cmd output inherited; minerr output inherited; scale output inherited; cvd_actual output inherited; err_thresh input inherited; rcs_use_in input inherited
function [rcs_cmd, minerr, scale, cvd_actual] = rcs_alloc(Bmat, wght_cv, ulim, llim, cvd_des, err_thresh, rcs_use_in)

rcs_quant = 0;
scale = 1;

nrcs = size(Bmat,2);


if(nrcs == 6)
    % assume fake RCS
    gang_pos = [0 0 0; 0 0 0; 1 1 0; 1 0 0; 0 0 1; 0 1 0];
    gang_neg = [1 1 0; 0 0 1; 0 0 0; 0 1 0; 0 0 0; 1 0 0];

    gain_factor = 1./diag(Bmat*gang_pos);
    rcs_cmd = gang_neg*(gain_factor.*max(0,-cvd_des)) + gang_pos*(gain_factor.*max(0,cvd_des));
    if(rcs_quant > 0)
        rcs_cmd = round(rcs_cmd/rcs_quant)*rcs_quant;
    end
    rcs_cmd = max(min(rcs_cmd,ulim),llim);
    cvd_actual = Bmat*rcs_cmd;
    minerr = norm(cvd_actual - cvd_des);
    
    return
end

rcs_cmd = llim;
cvd_actual = Bmat*rcs_cmd; 
minerr = norm((cvd_actual - cvd_des).*wght_cv);

if(minerr <= err_thresh)
    return
end

Bmat = diag(wght_cv)*Bmat;
cvd_des = wght_cv.*cvd_des;

scale_trial = 1;
normsq_cvd_trial = 0;

powersof2 = 2.^[0:nrcs-1];
bllim = uint32(powersof2*llim);
bulim = uint32(powersof2*ulim);
rcs_use_all = uint32([1:2^nrcs-1]');
rcs_use_tmp = bitor(rcs_use_all,uint32(bllim));
rcs_use_tmp = bitand(rcs_use_tmp,uint32(bulim));
rcs_use = rcs_use_in.*eq(rcs_use_tmp,rcs_use_all);

if(~any(rcs_use))
    return
end

for i = 1:length(rcs_use)
    
    if(~rcs_use(i))
        continue
    end
    
    rcson = double(bitget(uint32(i),1:nrcs))';
    cvd_trial = Bmat*rcson;
    
    % optional scaling
    if(0)
        scale_trial = dot(cvd_des,cvd_trial);
        if(scale_trial < 0)
            continue
        end
        
        normsq_cvd_trial = dot(cvd_trial,cvd_trial);
        if(normsq_cvd_trial <= scale_trial)
            scale_trial = 1;
        else
            scale_trial = dot(cvd_des,cvd_trial)/normsq_cvd_trial;
            cvd_trial = cvd_trial*scale_trial;
        end
    end
    
    cvd_ex = cvd_trial - cvd_des;
    err = norm(cvd_ex);
    if(err < minerr)
        scale = scale_trial;
        rcs_cmd = rcson*scale;
        minerr = err;
        cvd_actual = cvd_trial./wght_cv;
    end
end
